simulink model "dc_motor"  (R2018b)
settings: Solver=FixedStepAuto  StartTime=0.0  StopTime=SIM_TIME  FixedStep=STEP_SIZE  RelTol=1e-3
values from neighbouring files (symbols this model uses):
  Ce = Cm    (= 0.245)    [diploma_dc_motor.m]
  Cm = M_rated / I_rated    (= 0.245)    [diploma_dc_motor.m]
  DESIRED_SPEED = 0.15    [diploma_dc_motor.m]
  FZ_INSTEAD_PID = 0    [diploma_dc_motor.m]
  J = 0.00075    [diploma_dc_motor.m]
  k_p = 1    [diploma_dc_motor.m]
  k_vt = 0.05    [diploma_dc_motor.m]
  kd = 0.0001340    (= 0.000134)    [diploma_dc_motor.m]
  ki = 8.42    [diploma_dc_motor.m]
  kp = 0.0850    (= 0.085)    [diploma_dc_motor.m]
  L_ya = 0.01    [diploma_dc_motor.m]
  M_st = M_rated*1.5    (= 0.441)    [diploma_dc_motor.m]
  METER_TO_TICK = 1/0.0005167    (= 1935.3590091)    [diploma_dc_motor.m]
  R_ya = (U - Ce*w_rated)/I_rated    (= 5.36305555556)    [diploma_dc_motor.m]
  RPM_TO_TPS = 200/60    (= 3.33333333333)    [diploma_dc_motor.m]
  TICK_TO_METER = 0.0005167    [diploma_dc_motor.m]
  U = 9    [diploma_dc_motor.m]
libraries: fuzblock x1, simulink x1
settings Model: Creator=nex-lin  LastModifiedBy=nex-lin
settings SolverCC: ZeroCrossAlgorithm=Adaptive

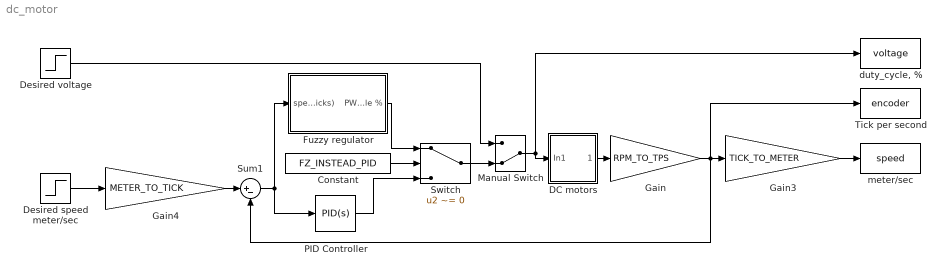
== system dc_motor ==
  Constant : Constant  Value=FZ_INSTEAD_PID
  DC motors : Subsystem
  Desired speed meter/sec : Step  Time=0  After=DESIRED_SPEED  SampleTime=0
  "Desired voltage " : Step  Time=0  After=U  SampleTime=0
  Fuzzy regulator : Subsystem
  Gain : Gain  Gain=RPM_TO_TPS
  Gain3 : Gain  Gain=TICK_TO_METER
  Gain4 : Gain  Gain=METER_TO_TICK
  Manual Switch : ManualSwitch  CurrentSetting=0
  PID Controller : simulink/Continuous/PID Controller  Controller=PID  Form=Parallel  TimeDomain=Continuous-time  SampleTime=-1  IntegratorMethod=Forward Euler  FilterMethod=Forward Euler  ControllerParametersSource=internal  P=kp  I=ki  D=kd  UseFilter=on  N=100  TunerSelectOption=Transfer Function Based (PID Tuner App)  InitialConditionSource=internal  InitialConditionForIntegrator=0  InitialConditionForFilter=0  DifferentiatorICPrevScaledInput=0  ExternalReset=none  TrackingMode=off  Kt=1  LimitOutput=off  UpperSaturationLimit=inf  LowerSaturationLimit=-inf  LinearizeAsGain=on  AntiWindupMode=none  Kb=1  POutMin=[]  POutMax=[]  IOutMin=[]  IOutMax=[]  DOutMin=[]  DOutMax=[]  NOutMin=[]  NOutMax=[]  SumOutMin=[]  SumOutMax=[]  SaturationOutMin=[]  SaturationOutMax=[]  PParamMin=[]  PParamMax=[]  IParamMin=[]  IParamMax=[]  DParamMin=[]  DParamMax=[]  NParamMin=[]  NParamMax=[]  KbParamMin=[]  KbParamMax=[]  KtParamMin=[]  KtParamMax=[]  KbOutMin=[]  KbOutMax=[]  KtOutMin=[]  KtOutMax=[]  IntegratorOutMin=[]  IntegratorOutMax=[]  FilterOutMin=[]  FilterOutMax=[]  SumI1OutMin=[]  SumI1OutMax=[]  SumI2OutMin=[]  SumI2OutMax=[]  SumI3OutMin=[]  SumI3OutMax=[]  SumI4OutMin=[]  SumI4OutMax=[]  SumDOutMin=[]  SumDOutMax=[]  DifferentiatorOutMin=[]  DifferentiatorOutMax=[]  FilterDiffOutCoefMin=[]  FilterDiffOutCoefMax=[]  ReciprocalOutMin=[]  ReciprocalOutMax=[]  SumDenOutMin=[]  SumDenOutMax=[]  SumNumOutMin=[]  SumNumOutMax=[]  DivideOutMin=[]  DivideOutMax=[]  IntegratorContinuousStateAttributes=''  IntegratorStateMustResolveToSignalObject=off  IntegratorRTWStateStorageClass=Auto  FilterContinuousStateAttributes=''  FilterStateMustResolveToSignalObject=off  FilterRTWStateStorageClass=Auto  ParallelPVariant=InternalParameters  IdealPVariant=Disabled  IVariant=InternalParameters  DVariant=InternalParameters  IntegratorVariant=Continuous  SatVariant=Disabled  AWVariant=Passthrough  PCopyVariant=Disabled  TRVariant=Disabled  FdbkBlocksVariant=Forward  IdealPFdbkVariant=Disabled  SatFdbkVariant=Disabled  DerivativeFilterVariant=ContFilter  NVariant=InternalParameters  NCopyVariant=Disabled  FilterICVariant=InternalICsFilter  IntegratorICVariant=InternalICs  ExternalResetVariant=Disabled  TRSumVariant=Passthrough  SumFdbkVariant=Disabled  SumVariant=Sum_PID
  Sum1 : Sum  Inputs=|+-
  Switch : Switch  Criteria=u2 ~= 0
  "Tick per second " : ToWorkspace  VariableName=encoder  SaveFormat=Structure With Time  SampleTime=-1
  "duty_cycle, %" : ToWorkspace  VariableName=voltage  SaveFormat=Structure With Time  SampleTime=-1
  meter/sec : ToWorkspace  VariableName=speed  SaveFormat=Structure With Time  SampleTime=-1
  wires:
  DC motors/1(Out1) -> Gain/1
  Gain/1 -> Sum1/2, "Tick per second "/1, Gain3/1
  Manual Switch/1 -> DC motors/1(In1), "duty_cycle, %"/1
  "Desired voltage "/1 -> Manual Switch/1
  Gain3/1 -> meter/sec/1
  Desired speed meter/sec/1 -> Gain4/1
  Sum1/1 -> PID Controller/1, Fuzzy regulator/1(speed difference (in Enc. Ticks))
  Gain4/1 -> Sum1/1
  Fuzzy regulator/1("PWM, duty cycle %") -> Switch/1
  Switch/1 -> Manual Switch/2
  Constant/1 -> Switch/2
  PID Controller/1 -> Switch/3

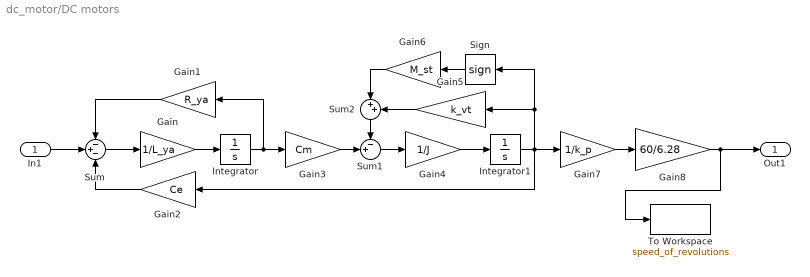
== system dc_motor/DC motors ==
  In1 : Inport
  Gain : Gain  Gain=1/L_ya
  Gain1 : Gain  Gain=R_ya
  Gain2 : Gain  Gain=Ce
  Gain3 : Gain  Gain=Cm
  Gain4 : Gain  Gain=1/J
  Gain5 : Gain  Gain=k_vt
  Gain6 : Gain  Gain=M_st
  Gain7 : Gain  Gain=1/k_p
  Gain8 : Gain  Gain=60/6.28
  Integrator : Integrator
  Integrator1 : Integrator
  Sign : Signum
  Sum : Sum  Inputs=-+-
  Sum1 : Sum  Inputs=-+|
  Sum2 : Sum  Inputs=|++
  To Workspace : ToWorkspace  VariableName=speed_of_revolutions  SaveFormat=Structure With Time  SampleTime=-1
  Out1 : Outport
  wires:
  Gain4/1 -> Integrator1/1
  Sum2/1 -> Sum1/1
  Gain/1 -> Integrator/1
  In1/1 -> Sum/2
  Sum/1 -> Gain/1
  Gain6/1 -> Sum2/1
  Sum1/1 -> Gain4/1
  Integrator1/1 -> Gain2/1, Sign/1, Gain5/1, Gain7/1
  Integrator/1 -> Gain1/1, Gain3/1
  Gain5/1 -> Sum2/2
  Gain7/1 -> Gain8/1
  Gain3/1 -> Sum1/2
  Sign/1 -> Gain6/1
  Gain8/1 -> Out1/1, To Workspace/1
  Gain1/1 -> Sum/1
  Gain2/1 -> Sum/3

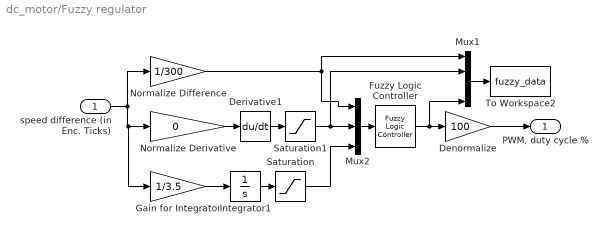
== system dc_motor/Fuzzy regulator ==
  speed difference (in Enc. Ticks) : Inport
  Denormalize : Gain  Gain=100
  Derivative1 : Derivative
  Fuzzy Logic Controller : fuzblock/Fuzzy Logic  Controller  FIS=fuzzy_regulator  OutputSampleNumber=101  DataType=double  FuzzifiedInputs=off  RuleFiringStrengths=off  RuleOutputs=off  AggregatedOutputs=off  SimulateUsing=Interpreted execution  OutOfRangeInputValueMessage=warning  NoRuleFiredMessage=warning  EmptyOutputFuzzySetMessage=warning
  Gain for Integrator : Gain  Gain=1/3.5
  Integrator1 : Integrator
  Mux1 : Mux
  Mux2 : Mux  Inputs=3
  Normalize Derivative : Gain  Gain=0
  Normalize Difference : Gain  Gain=1/300
  Saturation : Saturate  UpperLimit=1  LowerLimit=-1
  Saturation1 : Saturate  UpperLimit=0  LowerLimit=0
  To Workspace2 : ToWorkspace  VariableName=fuzzy_data  SaveFormat=Structure With Time  SampleTime=-1
  "PWM, duty cycle %" : Outport
  wires:
  Mux1/1 -> To Workspace2/1
  Mux2/1 -> Fuzzy Logic Controller/1
  speed difference (in Enc. Ticks)/1 -> Gain for Integrator/1, Normalize Derivative/1, Normalize Difference/1
  Derivative1/1 -> Saturation1/1
  Integrator1/1 -> Saturation/1
  Saturation1/1 -> Mux2/2, Mux1/2
  Fuzzy Logic Controller/1 -> Denormalize/1, Mux1/4
  Normalize Derivative/1 -> Derivative1/1
  Gain for Integrator/1 -> Integrator1/1
  Normalize Difference/1 -> Mux1/1, Mux2/1
  Denormalize/1 -> "PWM, duty cycle %"/1
  Saturation/1 -> Mux2/3
